simulink model "flow_circuit"  (R2021a)
settings: Solver=VariableStepAuto  StartTime=0.0  StopTime=10.0  RelTol=1e-3  AbsTol=1e-3
settings Model: Creator=ialak  LastModifiedBy=ialak
settings SolverCC: AutoScaleAbsTol=off  AlgebraicLoopSolver=TrustRegion
settings DataIOCC: LoggingToFile=on
settings DebuggingCC: SymbolicDimsDataTypeCodeGenerationDiagnostic=none  SFMachineParentedDataDiag=warning
settings SFSimCC: CustomCodeUndefinedFunction=UseInterfaceOnly
settings SimscapeCC: SimscapeLogType=all  SimscapeLogSimulationStatistics=on  SimscapeLogDataHistory=10000

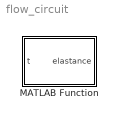
== system flow_circuit ==
  MATLAB Function : MATLAB Function  TreatAsAtomicUnit=on

== matlab function flow_circuit/MATLAB Function ==
  data: t input; elastance output
function elastance = fcn(t)
T = 1;
T_pwb = 0.91;
T_pww = 0.09;
E_la_max = 0.25;
E_la_min = 0.15;

t = mod(t,T);

if t < T_pwb
    elastance = E_la_min;
elseif t < (T_pwb + T_pww) && t >= T_pwb
    elastance = E_la_min + (E_la_max - E_la_min)/2 * (1-cos(((t-T_pwb)/T_pww)*2*pi));
else
    elastance = E_la_min;
end
elastance = t;
